simulink model "circuit_Rasp_2"  (R2018b)
settings: Solver=VariableStepAuto  StartTime=0.0  StopTime=10.0  RelTol=1e-3
libraries: pe_lib x20, fl_lib x13
settings Model: Creator=giovannirenda  LastModifiedBy=giovannirenda
settings DebuggingCC: LibraryContextMissingDiagnostic=none
settings SFSimCC: SimUseLocalCustomCode=off
settings RTWCC: RTWUseLocalCustomCode=off

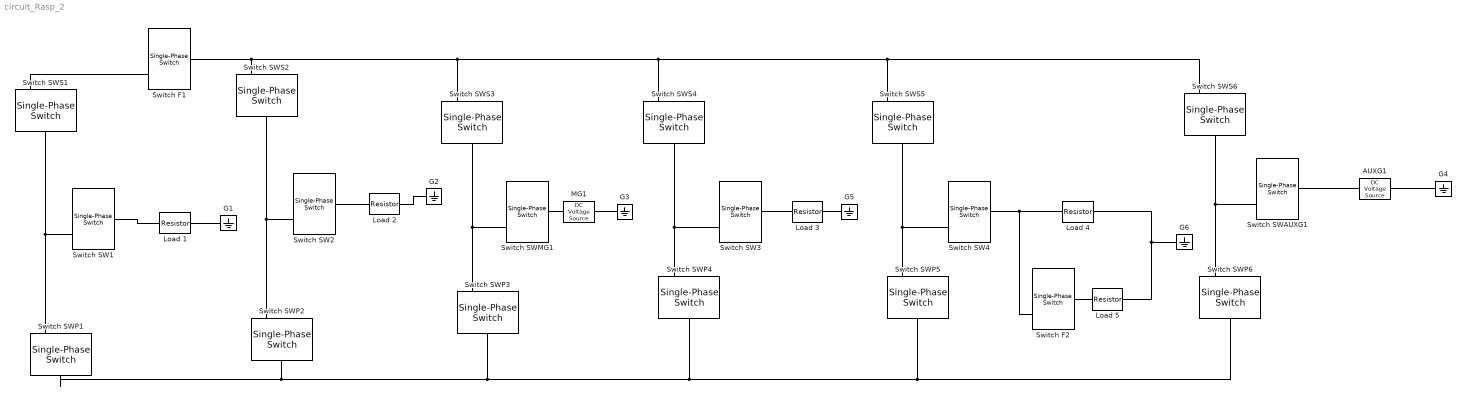
== system circuit_Rasp_2 ==
  AUXG1 : fl_lib/Electrical/Electrical Sources/DC Voltage Source  v0=3.3 V
  G{1..6} (6 alike) : fl_lib/Electrical/Electrical Elements/Electrical Reference
  Load 1 : fl_lib/Electrical/Electrical Elements/Resistor  R=12.7 Ohm  i_specify=off  i_priority=None  i=0 A  i_nominal_specify=off  i_nominal_unit=A  i_nominal_value=1  v_specify=off  v_priority=None  v=0 V  v_nominal_specify=off  v_nominal_unit=V  v_nominal_value=1
  Load 2 : fl_lib/Electrical/Electrical Elements/Resistor  R=12.7 Ohm  i_specify=off  i_priority=None  i=0 A  i_nominal_specify=off  i_nominal_unit=A  i_nominal_value=1  v_specify=off  v_priority=None  v=0 V  v_nominal_specify=off  v_nominal_unit=V  v_nominal_value=1
  Load 3 : fl_lib/Electrical/Electrical Elements/Resistor  R=91.67 Ohm  i_specify=off  i_priority=None  i=0 A  i_nominal_specify=off  i_nominal_unit=A  i_nominal_value=1  v_specify=off  v_priority=None  v=0 V  v_nominal_specify=off  v_nominal_unit=V  v_nominal_value=1
  Load 4 : fl_lib/Electrical/Electrical Elements/Resistor  R=91.67 Ohm  i_specify=off  i_priority=None  i=0 A  i_nominal_specify=off  i_nominal_unit=A  i_nominal_value=1  v_specify=off  v_priority=None  v=0 V  v_nominal_specify=off  v_nominal_unit=V  v_nominal_value=1
  Load 5 : fl_lib/Electrical/Electrical Elements/Resistor  R=91.67 Ohm  i_specify=off  i_priority=None  i=0 A  i_nominal_specify=off  i_nominal_unit=A  i_nominal_value=1  v_specify=off  v_priority=None  v=0 V  v_nominal_specify=off  v_nominal_unit=V  v_nominal_value=1
  MG1 : fl_lib/Electrical/Electrical Sources/DC Voltage Source  v0=3.3 V
  Switch F1 : pe_lib/Switches & Breakers/Fundamental Components/Single-Phase Switch  R_closed=0.001 Ohm  G_open=1e-6 1/Ohm  threshold=0 V
      settings: SourceProductName=Simscape Electrical  SourceProductBaseCode=PS
  Switch F2 : pe_lib/Switches & Breakers/Fundamental Components/Single-Phase Switch  R_closed=0.001 Ohm  G_open=1e-6 1/Ohm  threshold=0 V
      settings: SourceProductName=Simscape Electrical  SourceProductBaseCode=PS
  Switch SW{1..4} (4 alike) : pe_lib/Switches & Breakers/Fundamental Components/Single-Phase Switch  R_closed=0.001 Ohm  G_open=1e-6 1/Ohm  threshold=0 V
      settings: SourceProductName=Simscape Electrical  SourceProductBaseCode=PS
  Switch SWAUXG1 : pe_lib/Switches & Breakers/Fundamental Components/Single-Phase Switch  R_closed=0.001 Ohm  G_open=1e-6 1/Ohm  threshold=0 V
      settings: SourceProductName=Simscape Electrical  SourceProductBaseCode=PS
  Switch SWMG1 : pe_lib/Switches & Breakers/Fundamental Components/Single-Phase Switch  R_closed=0.001 Ohm  G_open=1e-6 1/Ohm  threshold=0 V
      settings: SourceProductName=Simscape Electrical  SourceProductBaseCode=PS
  Switch SWP{1..6} (6 alike) : pe_lib/Switches & Breakers/Fundamental Components/Single-Phase Switch  R_closed=0.001 Ohm  G_open=1e-6 1/Ohm  threshold=0 V
      settings: SourceProductName=Simscape Electrical  SourceProductBaseCode=PS
  Switch SWS{1..6} (6 alike) : pe_lib/Switches & Breakers/Fundamental Components/Single-Phase Switch  R_closed=0.001 Ohm  G_open=1e-6 1/Ohm  threshold=0 V
      settings: SourceProductName=Simscape Electrical  SourceProductBaseCode=PS
  connections:
  Switch SW1/LConn2 -- Switch SWP1/LConn2 -- Switch SWS1/RConn1
  Load 1/RConn1 -- G1/LConn1
  G3/LConn1 -- MG1/RConn1
  Switch SWS6/LConn2 -- Switch SWS4/LConn2 -- Switch SWS3/LConn2 -- Switch SWS2/LConn2 -- Switch F1/RConn1 -- Switch SWS5/LConn2
  Switch SWP1/RConn1 -- Switch SWP2/RConn1 -- Switch SWP6/RConn1 -- Switch SWP5/RConn1 -- Switch SWP4/RConn1 -- Switch SWP3/RConn1
  Switch SWS1/LConn2 -- Switch F1/LConn2
  MG1/LConn1 -- Switch SWMG1/RConn1
  Load 1/LConn1 -- Switch SW1/RConn1
  AUXG1/RConn1 -- G4/LConn1
  AUXG1/LConn1 -- Switch SWAUXG1/RConn1
  Switch SWS2/RConn1 -- Switch SW2/LConn2 -- Switch SWP2/LConn2
  Switch SWMG1/LConn2 -- Switch SWS3/RConn1 -- Switch SWP3/LConn2
  Switch SWP4/LConn2 -- Switch SWS4/RConn1 -- Switch SW3/LConn2
  G5/LConn1 -- Load 3/RConn1
  Switch SW3/RConn1 -- Load 3/LConn1
  Switch SWP5/LConn2 -- Switch SWS5/RConn1 -- Switch SW4/LConn2
  G6/LConn1 -- Load 4/RConn1 -- Load 5/RConn1
  Switch SWAUXG1/LConn2 -- Switch SWS6/RConn1 -- Switch SWP6/LConn2
  Load 2/RConn1 -- G2/LConn1
  Load 2/LConn1 -- Switch SW2/RConn1
  Switch SW4/RConn1 -- Load 4/LConn1 -- Switch F2/LConn2
  Switch F2/RConn1 -- Load 5/LConn1
